simulink model "simulazione_005_s"  (R2016b)
settings: Solver=ode4  StartTime=0.0  StopTime=t_sim  FixedStep=step  RelTol=1e-3
values from neighbouring files (symbols this model uses):
  delta_x = -1    [simulazione_005_init.m]
  movement_lower_limit = -movement_upper_limit    [simulazione_005_init.m]
  movement_upper_limit = [2*pi; 2*pi; 2*pi; 2*pi; 2*pi; 2*pi]    [simulazione_005_init.m]
  p_init = direct_kinematic(q_init)    [simulazione_005_init.m]
  q_init = [0; 0; 0; 0; 0; 0]    [simulazione_005_init.m]
  t_exe = 2    [simulazione_005_init.m]
  velocity_lower_limit = -velocity_upper_limit    [simulazione_005_init.m]
  velocity_upper_limit = [2*pi/3; 2*pi/3; pi; pi; pi; pi]    [simulazione_005_init.m]
settings Model: Creator=IBM  LastModifiedBy=IBM

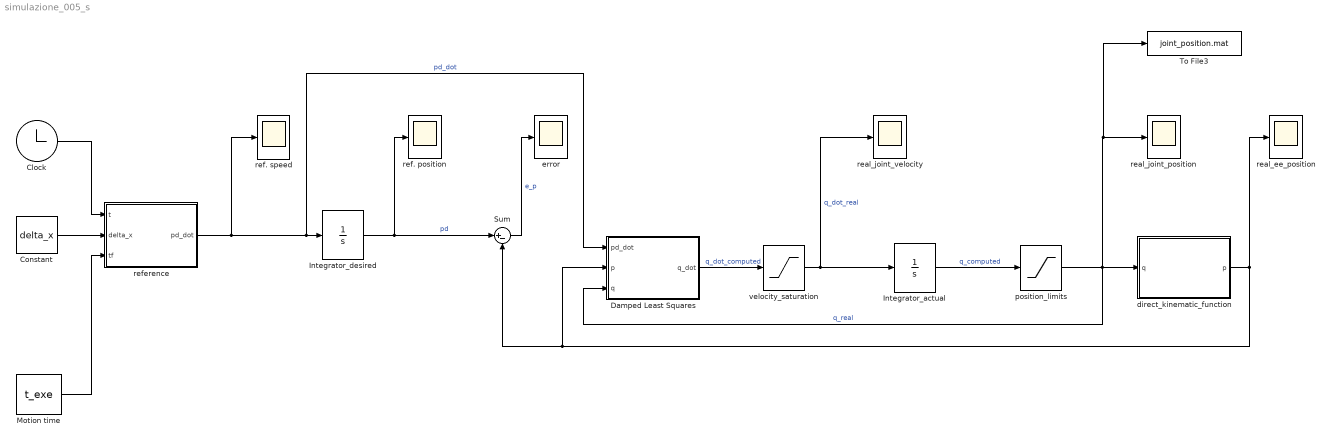
== system simulazione_005_s ==
  Clock : Clock
  Constant : Constant  Value=delta_x
  "Damped Least Squares " : MATLAB Function  TreatAsAtomicUnit=on
  Integrator_actual : Integrator  InitialCondition=q_init
  Integrator_desired : Integrator  InitialCondition=p_init
  Motion time : Constant  Value=t_exe
  Sum : Sum  Inputs=|+-
  To File3 : ToFile  Filename=joint_position.mat  MatrixName=q
  direct_kinematic_function : MATLAB Function  TreatAsAtomicUnit=on
  error : Scope
  position_limits : Saturate  UpperLimit=movement_upper_limit  LowerLimit=movement_lower_limit
  real_ee_position : Scope
  real_joint_position : Scope
  real_joint_velocity : Scope
  ref. position : Scope
  ref. speed : Scope
  reference : MATLAB Function  TreatAsAtomicUnit=on
  velocity_saturation : Saturate  UpperLimit=velocity_upper_limit  LowerLimit=velocity_lower_limit
  wires:
  Clock/1 -> reference/1(t)
  Integrator_desired/1 -> ref. position/1, Sum/1  "pd"
  Motion time/1 -> reference/3(tf)
  Sum/1 -> error/1  "e_p"
  Integrator_actual/1 -> position_limits/1  "q_computed"
  direct_kinematic_function/1(p) -> real_ee_position/1, "Damped Least Squares "/2(p), Sum/2
  Constant/1 -> reference/2(delta_x)
  reference/1(pd_dot) -> ref. speed/1, "Damped Least Squares "/1(pd_dot), Integrator_desired/1  "pd_dot"
  position_limits/1 -> To File3/1, real_joint_position/1, "Damped Least Squares "/3(q), direct_kinematic_function/1(q)  "q_real"
  "Damped Least Squares "/1(q_dot) -> velocity_saturation/1  "q_dot_computed"
  velocity_saturation/1 -> real_joint_velocity/1, Integrator_actual/1  "q_dot_real"

== matlab function simulazione_005_s/Damped Least Squares  ==
  data: pd_dot input; p input; q_dot output; q input
function q_dot = DLS(pd_dot, p, q)
    
    Jg = geometric_jacobian(q);
    Ja = analytic_jacobian(Jg, p);
    
    s = svd(Ja);
    sigma_th = 1/pi;
    sigma = s(6);
    lambda_max = 0.001;
    
    if sigma >= sigma_th 
        lambda = 0; 
    else
        lambda = lambda_max - lambda_max * sigma / sigma_th;
    end
    
    q_dot = transpose(Ja) * inv(Ja * transpose(Ja) + lambda * eye(6)) * pd_dot;
    
end

== matlab function simulazione_005_s/reference ==
  data: t input; delta_x input; pd_dot output; tf input
function pd_dot = reference(t, delta_x, tf)

    pd_dot = linear_reference(t, delta_x, tf);
    
end

== matlab function simulazione_005_s/direct_kinematic_function ==
  data: q input; p output
function p = dkf(q)

    p = direct_kinematic(q);
